simulink model "anti"  (R2020a)
settings: Solver=VariableStepAuto  StartTime=0.0  StopTime=10.0  RelTol=1e-3
settings Model: Creator=Ali  LastModifiedBy=Ali

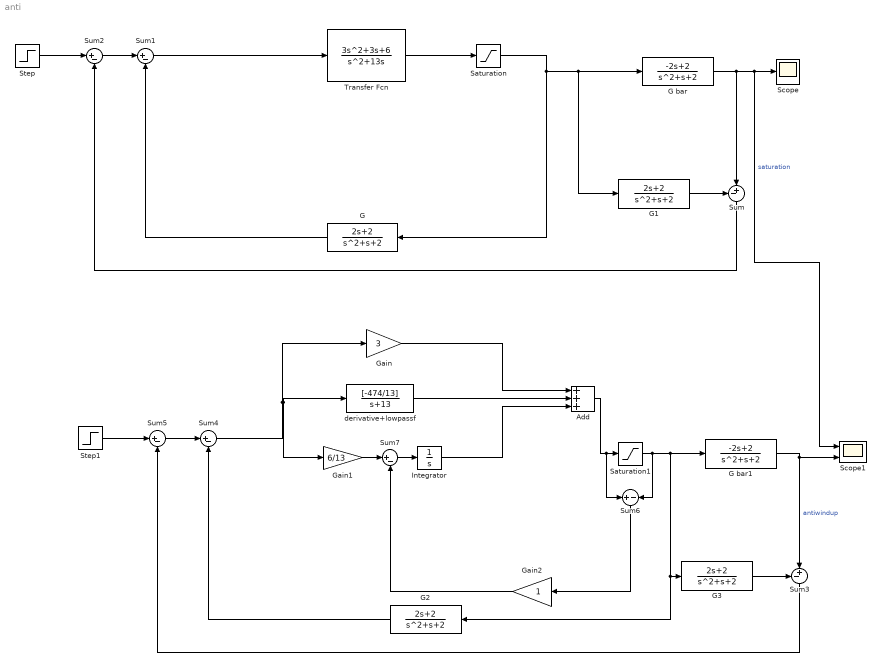
== system anti ==
  Add : Sum  Inputs=+++
  G{,1..3} (4 alike) : TransferFcn  Numerator=[2 2]  Denominator=[1 1 2]
  G bar : TransferFcn  Numerator=[-2 2]  Denominator=[1 1 2]
  G bar1 : TransferFcn  Numerator=[-2 2]  Denominator=[1 1 2]
  Gain : Gain  Gain=3
  Gain1 : Gain  Gain=6/13
  Gain2 : Gain
  Integrator : Integrator
  Saturation : Saturate  UpperLimit=1.5  LowerLimit=-1.5
  Saturation1 : Saturate  UpperLimit=1.5  LowerLimit=-1.5
  Scope : Scope
  Scope1 : Scope  NumInputPorts=2
  Step : Step  Time=0  SampleTime=0
  Step1 : Step  Time=0  SampleTime=0
  Sum : Sum  Inputs=-+|
  Sum{1..2,4..5,7} (5 alike) : Sum  Inputs=|+-
  Sum3 : Sum  Inputs=-+|
  Sum6 : Sum  Inputs=+-
  Transfer Fcn : TransferFcn  Numerator=[3 3 6]  Denominator=[1 13 0]
  derivative+lowpassf : TransferFcn  Numerator=[-474/13]  Denominator=[1 13]
  wires:
  Transfer Fcn/1 -> Saturation/1
  G bar/1 -> Sum/2, Scope1/1, Scope/1  "saturation"
  G1/1 -> Sum/1
  G/1 -> Sum1/2
  Sum2/1 -> Sum1/1
  Sum/1 -> Sum2/2
  Step/1 -> Sum2/1
  Gain1/1 -> Sum7/1
  derivative+lowpassf/1 -> Add/2
  Gain/1 -> Add/1
  Sum4/1 -> Gain/1, Gain1/1, derivative+lowpassf/1
  Integrator/1 -> Add/3
  Sum1/1 -> Transfer Fcn/1
  Saturation/1 -> G/1, G1/1, G bar/1
  Sum3/1 -> Sum5/2
  G bar1/1 -> Sum3/2, Scope1/2  "antiwindup"
  Sum5/1 -> Sum4/1
  G2/1 -> Sum4/2
  Step1/1 -> Sum5/1
  G3/1 -> Sum3/1
  Add/1 -> Sum6/1, Saturation1/1
  Saturation1/1 -> Sum6/2, G2/1, G3/1, G bar1/1
  Gain2/1 -> Sum7/2
  Sum6/1 -> Gain2/1
  Sum7/1 -> Integrator/1
